simulink model "robot_assembly_backup_oke"  (R2016a)
settings: Solver=VariableStepAuto  StartTime=0.0  StopTime=inf  RelTol=1e-3
values from neighbouring files (symbols this model uses):
  m = size(X, 1)    [polyfitn.m]
undefined symbols (not defined in the file or in its folder): Khop3, Khop_1, Khop_2, Khop_4, Khop_5, Khop_6, robot_assembly, RootGround, RootPart
libraries: mblibv1 x21, simulink x5
settings Model: Creator=Hieu  LastModifiedBy=Hieu
settings GRTTargetCC: GeneratePreprocessorConditionals=Use local settings
settings SimMechanicsCC: VisOnUpdateDiagram=on  VisDuringSimulation=on

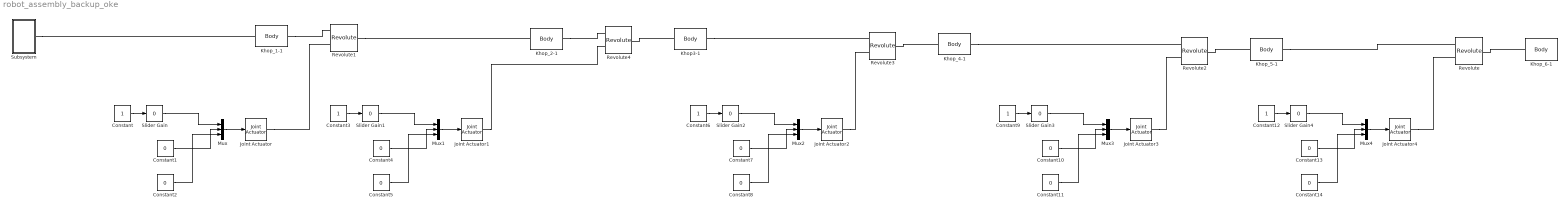
== system robot_assembly_backup_oke ==
  Constant{,3,6,9,12} (5 alike) : Constant
  Constant{1..2,4..5,7..8,10..11,13..14} (10 alike) : Constant  Value=0
  Joint Actuator{,1..4} (5 alike) : mblibv1/Sensors &  Actuators/Joint Actuator  UpdateFromCAD=off  PhysicalDomain=Mechanical  PortType=blob  ActuationStyle=Motion  AngleUnits=deg  ArcVelocityUnits=deg/s  ArcAccelerationUnits=deg/s^2  CoordPositionUnits=m  VelocityUnits=m/s  AccelerationUnits=m/s^2  ForceUnits=N  TorqueUnits=N*m  ActiveIO=on  Width=3  DialogClass=MechanicalActuatorBlock  Primitive=R1  ReferenceFrame=Absolute (World)
  Khop3-1 : mblibv1/Bodies/Body  LConnTagsString=CS3  RConnTagsString=CS2  UpdateFromCAD=on  PMImportedID=Khop3-1  DialogClass=MechanicalBodyBlock  Mass=43.6159  MassUnits=kg  InertiaUnits=kg*m^2  Inertia=[1.17816,2.48356e-09,1.21289e-08;2.48356e-09,0.116751,-0.0778152;1.21289e-08,-0.0778152,1.13755]  Shape=Cylinder  ShapeDims=[1 1]  ShapeUnits=m  ShapeUse=false  Density=1  DensityUnits=kg/m^3  DensityUse=false  GraphicsMode=GFXFILE  GraphicsFileName=robot_assembly - Khop3-1.STL  BodyColorSelMode=COLORPALETTE  BodyColor=[0.776471;0.756863;0.737255]  AttachedToCS=CS1  CG=Right$CG$[0.1867 1.03234 0.317413]$WORLD$WORLD$m$[0.332848 -0.650354 -0.682826;0.890188 0.455594 0;0.311091 -0.607844 0.730581]$3x3 Transform$rad$WORLD$false$Khop3-1::CG(AUTOGEN)  WorkingFrames=Right$CS1$[0.352941 0.944212 0.39173]$WORLD$WORLD$m$[0.332848 -0.650354 -0.682826;0.890188 0.455594 0;0.311091 -0.607844 0.730581]$3x3 Transform$rad$WORLD$false$Khop3-1::CS1(AUTOGEN)#Right$CS2$[-0.028645 1.11825 0.301997]$WORLD$WORLD$m$[1 0 0;0 1 0;0 0 1]$3x3 Transform$rad$WORLD$true$Khop3-1:-:Khop_4-1::Khop3-1(AUTOGEN)#Left$CS3$[0.281245 0.944212 0.468441]$WORLD$WORLD$m$[1 0 0;0 1 0;0 0 1]$3x3 Transform$rad$WORLD$true$Khop3-1:-:Khop_2-1::Khop3-1(AUTOGEN)  CGPos=[0.1867 1.03234 0.317413]  CGRot=[0.332848 -0.650354 -0.682826;0.890188 0.455594 0;0.311091 -0.607844 0.730581]  CS0Pos=[]  CS0Rot=[]  CS1Pos=[0.352941 0.944212 0.39173]  CS1Rot=[0.332848 -0.650354 -0.682826;0.890188 0.455594 0;0.311091 -0.607844 0.730581]  CS2Pos=[-0.028645 1.11825 0.301997]  CS2Rot=[1 0 0;0 1 0;0 0 1]  CS3Pos=[0.281245 0.944212 0.468441]  CS3Rot=[1 0 0;0 1 0;0 0 1]  CS4Pos=[]  CS4Rot=[]  CS5Pos=[]  CS5Rot=[]  CS6Pos=[]  CS6Rot=[]  CS7Pos=[]  CS7Rot=[]  CS8Pos=[]  CS8Rot=[]  CS9Pos=[]  CS9Rot=[]  CS10Pos=[]  CS10Rot=[]  CS11Pos=[]  CS11Rot=[]  CS12Pos=[]  CS12Rot=[]  CS13Pos=[]  CS13Rot=[]  CS14Pos=[]  CS14Rot=[]  CS15Pos=[]  CS15Rot=[]  CS16Pos=[]  CS16Rot=[]  CS17Pos=[]  CS17Rot=[]  CS18Pos=[]  CS18Rot=[]  CS19Pos=[]  CS19Rot=[]  CS20Pos=[]  CS20Rot=[]
  Khop_1-1 : mblibv1/Bodies/Body  LConnTagsString=CS2  RConnTagsString=CS3  UpdateFromCAD=on  PMImportedID=Khop_1-1  DialogClass=MechanicalBodyBlock  Mass=159.648  MassUnits=kg  InertiaUnits=kg*m^2  Inertia=[4.67506,0.0155226,1.62056e-06;0.0155226,1.87752,-4.14461e-06;1.62056e-06,-4.14461e-06,4.39981]  Shape=Cylinder  ShapeDims=[1 1]  ShapeUnits=m  ShapeUse=false  Density=1  DensityUnits=kg/m^3  DensityUse=false  GraphicsMode=GFXFILE  GraphicsFileName=robot_assembly - Khop_1-1.STL  BodyColorSelMode=COLORPALETTE  BodyColor=[0.054902;0.054902;0.054902]  AttachedToCS=CS1  CG=Right$CG$[0.24168 0.390199 0.514197]$WORLD$WORLD$m$[1 0 0;0 1 0;0 0 1]$3x3 Transform$rad$WORLD$false$Khop_1-1::CG(AUTOGEN)  WorkingFrames=Right$CS1$[0.238479 0.145212 0.514197]$WORLD$WORLD$m$[1 0 0;0 1 0;0 0 1]$3x3 Transform$rad$WORLD$false$Khop_1-1::CS1(AUTOGEN)#Left$CS2$[0.24168 0.390199 0.514197]$WORLD$WORLD$m$[1 0 0;0 1 0;0 0 1]$3x3 Transform$rad$WORLD$true$Khop_1-1:-:robot_assembly/RootPart::Khop_1-1(AUTOGEN)#Right$CS3$[0.238479 0.705212 0.514197]$WORLD$WORLD$m$[1 0 0;0 1 0;0 0 1]$3x3 Transform$rad$WORLD$true$Khop_1-1:-:Khop_2-1::Khop_1-1(AUTOGEN)  CGPos=[0.24168 0.390199 0.514197]  CGRot=[1 0 0;0 1 0;0 0 1]  CS0Pos=[]  CS0Rot=[]  CS1Pos=[0.238479 0.145212 0.514197]  CS1Rot=[1 0 0;0 1 0;0 0 1]  CS2Pos=[0.24168 0.390199 0.514197]  CS2Rot=[1 0 0;0 1 0;0 0 1]  CS3Pos=[0.238479 0.705212 0.514197]  CS3Rot=[1 0 0;0 1 0;0 0 1]  CS4Pos=[]  CS4Rot=[]  CS5Pos=[]  CS5Rot=[]  CS6Pos=[]  CS6Rot=[]  CS7Pos=[]  CS7Rot=[]  CS8Pos=[]  CS8Rot=[]  CS9Pos=[]  CS9Rot=[]  CS10Pos=[]  CS10Rot=[]  CS11Pos=[]  CS11Rot=[]  CS12Pos=[]  CS12Rot=[]  CS13Pos=[]  CS13Rot=[]  CS14Pos=[]  CS14Rot=[]  CS15Pos=[]  CS15Rot=[]  CS16Pos=[]  CS16Rot=[]  CS17Pos=[]  CS17Rot=[]  CS18Pos=[]  CS18Rot=[]  CS19Pos=[]  CS19Rot=[]  CS20Pos=[]  CS20Rot=[]
  Khop_2-1 : mblibv1/Bodies/Body  LConnTagsString=CS2  RConnTagsString=CS3  UpdateFromCAD=on  PMImportedID=Khop_2-1  DialogClass=MechanicalBodyBlock  Mass=96.4098  MassUnits=kg  InertiaUnits=kg*m^2  Inertia=[1.36159,-0.133561,-9.98407e-05;-0.133561,0.612029,-6.13842e-05;-9.98407e-05,-6.13842e-05,1.31785]  Shape=Cylinder  ShapeDims=[1 1]  ShapeUnits=m  ShapeUse=false  Density=1  DensityUnits=kg/m^3  DensityUse=false  GraphicsMode=GFXFILE  GraphicsFileName=robot_assembly - Khop_2-1.STL  BodyColorSelMode=COLORPALETTE  BodyColor=[0.94902;0.352941;0.0666667]  AttachedToCS=CS1  CG=Right$CG$[0.224023 0.863366 0.529676]$WORLD$WORLD$m$[-0.682826 0 -0.730581;0 1 0;0.730581 0 -0.682826]$3x3 Transform$rad$WORLD$false$Khop_2-1::CG(AUTOGEN)  WorkingFrames=Right$CS1$[0.238479 0.705212 0.514197]$WORLD$WORLD$m$[-0.682826 0 -0.730581;0 1 0;0.730581 0 -0.682826]$3x3 Transform$rad$WORLD$false$Khop_2-1::CS1(AUTOGEN)#Left$CS2$[0.238479 0.705212 0.514197]$WORLD$WORLD$m$[1 0 0;0 1 0;0 0 1]$3x3 Transform$rad$WORLD$true$Khop_1-1:-:Khop_2-1::Khop_2-1(AUTOGEN)#Right$CS3$[0.281245 0.944212 0.468441]$WORLD$WORLD$m$[1 0 0;0 1 0;0 0 1]$3x3 Transform$rad$WORLD$true$Khop3-1:-:Khop_2-1::Khop_2-1(AUTOGEN)  CGPos=[0.224023 0.863366 0.529676]  CGRot=[-0.682826 0 -0.730581;0 1 0;0.730581 0 -0.682826]  CS0Pos=[]  CS0Rot=[]  CS1Pos=[0.238479 0.705212 0.514197]  CS1Rot=[-0.682826 0 -0.730581;0 1 0;0.730581 0 -0.682826]  CS2Pos=[0.238479 0.705212 0.514197]  CS2Rot=[1 0 0;0 1 0;0 0 1]  CS3Pos=[0.281245 0.944212 0.468441]  CS3Rot=[1 0 0;0 1 0;0 0 1]  CS4Pos=[]  CS4Rot=[]  CS5Pos=[]  CS5Rot=[]  CS6Pos=[]  CS6Rot=[]  CS7Pos=[]  CS7Rot=[]  CS8Pos=[]  CS8Rot=[]  CS9Pos=[]  CS9Rot=[]  CS10Pos=[]  CS10Rot=[]  CS11Pos=[]  CS11Rot=[]  CS12Pos=[]  CS12Rot=[]  CS13Pos=[]  CS13Rot=[]  CS14Pos=[]  CS14Rot=[]  CS15Pos=[]  CS15Rot=[]  CS16Pos=[]  CS16Rot=[]  CS17Pos=[]  CS17Rot=[]  CS18Pos=[]  CS18Rot=[]  CS19Pos=[]  CS19Rot=[]  CS20Pos=[]  CS20Rot=[]
  Khop_4-1 : mblibv1/Bodies/Body  LConnTagsString=CS3  RConnTagsString=CS2  UpdateFromCAD=on  PMImportedID=Khop_4-1  DialogClass=MechanicalBodyBlock  Mass=91.2451  MassUnits=kg  InertiaUnits=kg*m^2  Inertia=[6.24377,0,0.707353;0,6.5607,0;0.707353,0,0.475899]  Shape=Cylinder  ShapeDims=[1 1]  ShapeUnits=m  ShapeUse=false  Density=1  DensityUnits=kg/m^3  DensityUse=false  GraphicsMode=GFXFILE  GraphicsFileName=robot_assembly - Khop_4-1.STL  BodyColorSelMode=COLORPALETTE  BodyColor=[0.776471;0.756863;0.737255]  AttachedToCS=CS1  CG=Right$CG$[-0.127156 1.13763 0.332657]$WORLD$WORLD$m$[-0.682826 0.259349 -0.682998;0 0.93487 0.35499;0.730581 0.242397 -0.638354]$3x3 Transform$rad$WORLD$false$Khop_4-1::CG(AUTOGEN)  WorkingFrames=Right$CS1$[-0.028645 1.11825 0.301997]$WORLD$WORLD$m$[-0.682826 0.259349 -0.682998;0 0.93487 0.35499;0.730581 0.242397 -0.638354]$3x3 Transform$rad$WORLD$false$Khop_4-1::CS1(AUTOGEN)#Right$CS2$[-0.370144 1.29574 -0.0171799]$WORLD$WORLD$m$[1 0 0;0 1 0;0 0 1]$3x3 Transform$rad$WORLD$true$Khop_4-1:-:Khop_5-1::Khop_4-1(AUTOGEN)#Left$CS3$[-0.028645 1.11825 0.301997]$WORLD$WORLD$m$[1 0 0;0 1 0;0 0 1]$3x3 Transform$rad$WORLD$true$Khop3-1:-:Khop_4-1::Khop_4-1(AUTOGEN)  CGPos=[-0.127156 1.13763 0.332657]  CGRot=[-0.682826 0.259349 -0.682998;0 0.93487 0.35499;0.730581 0.242397 -0.638354]  CS0Pos=[]  CS0Rot=[]  CS1Pos=[-0.028645 1.11825 0.301997]  CS1Rot=[-0.682826 0.259349 -0.682998;0 0.93487 0.35499;0.730581 0.242397 -0.638354]  CS2Pos=[-0.370144 1.29574 -0.0171799]  CS2Rot=[1 0 0;0 1 0;0 0 1]  CS3Pos=[-0.028645 1.11825 0.301997]  CS3Rot=[1 0 0;0 1 0;0 0 1]  CS4Pos=[]  CS4Rot=[]  CS5Pos=[]  CS5Rot=[]  CS6Pos=[]  CS6Rot=[]  CS7Pos=[]  CS7Rot=[]  CS8Pos=[]  CS8Rot=[]  CS9Pos=[]  CS9Rot=[]  CS10Pos=[]  CS10Rot=[]  CS11Pos=[]  CS11Rot=[]  CS12Pos=[]  CS12Rot=[]  CS13Pos=[]  CS13Rot=[]  CS14Pos=[]  CS14Rot=[]  CS15Pos=[]  CS15Rot=[]  CS16Pos=[]  CS16Rot=[]  CS17Pos=[]  CS17Rot=[]  CS18Pos=[]  CS18Rot=[]  CS19Pos=[]  CS19Rot=[]  CS20Pos=[]  CS20Rot=[]
  Khop_5-1 : mblibv1/Bodies/Body  LConnTagsString=CS3  RConnTagsString=CS2  UpdateFromCAD=on  PMImportedID=Khop_5-1  DialogClass=MechanicalBodyBlock  Mass=4.20495  MassUnits=kg  InertiaUnits=kg*m^2  Inertia=[0.00605149,-7.30355e-05,-2.13324e-09;-7.30355e-05,0.00377876,2.04521e-09;-2.13324e-09,2.04521e-09,0.00491242]  Shape=Cylinder  ShapeDims=[1 1]  ShapeUnits=m  ShapeUse=false  Density=1  DensityUnits=kg/m^3  DensityUse=false  GraphicsMode=GFXFILE  GraphicsFileName=robot_assembly - Khop_5-1.STL  BodyColorSelMode=COLORPALETTE  BodyColor=[0.776471;0.756863;0.737255]  AttachedToCS=CS1  CG=Right$CG$[-0.350069 1.29118 -0.0409774]$WORLD$WORLD$m$[-0.682826 -0.239308 0.690275;0 -0.944831 -0.327558;0.730581 -0.223665 0.645156]$3x3 Transform$rad$WORLD$false$Khop_5-1::CG(AUTOGEN)  WorkingFrames=Right$CS1$[-0.332589 1.29574 -0.0573619]$WORLD$WORLD$m$[-0.682826 -0.239308 0.690275;0 -0.944831 -0.327558;0.730581 -0.223665 0.645156]$3x3 Transform$rad$WORLD$false$Khop_5-1::CS1(AUTOGEN)#Right$CS2$[-0.363332 1.2485 -0.0484542]$WORLD$WORLD$m$[1 0 0;0 1 0;0 0 1]$3x3 Transform$rad$WORLD$true$Khop_5-1:-:Khop_6-1::Khop_5-1(AUTOGEN)#Left$CS3$[-0.370144 1.29574 -0.0171799]$WORLD$WORLD$m$[1 0 0;0 1 0;0 0 1]$3x3 Transform$rad$WORLD$true$Khop_4-1:-:Khop_5-1::Khop_5-1(AUTOGEN)  CGPos=[-0.350069 1.29118 -0.0409774]  CGRot=[-0.682826 -0.239308 0.690275;0 -0.944831 -0.327558;0.730581 -0.223665 0.645156]  CS0Pos=[]  CS0Rot=[]  CS1Pos=[-0.332589 1.29574 -0.0573619]  CS1Rot=[-0.682826 -0.239308 0.690275;0 -0.944831 -0.327558;0.730581 -0.223665 0.645156]  CS2Pos=[-0.363332 1.2485 -0.0484542]  CS2Rot=[1 0 0;0 1 0;0 0 1]  CS3Pos=[-0.370144 1.29574 -0.0171799]  CS3Rot=[1 0 0;0 1 0;0 0 1]  CS4Pos=[]  CS4Rot=[]  CS5Pos=[]  CS5Rot=[]  CS6Pos=[]  CS6Rot=[]  CS7Pos=[]  CS7Rot=[]  CS8Pos=[]  CS8Rot=[]  CS9Pos=[]  CS9Rot=[]  CS10Pos=[]  CS10Rot=[]  CS11Pos=[]  CS11Rot=[]  CS12Pos=[]  CS12Rot=[]  CS13Pos=[]  CS13Rot=[]  CS14Pos=[]  CS14Rot=[]  CS15Pos=[]  CS15Rot=[]  CS16Pos=[]  CS16Rot=[]  CS17Pos=[]  CS17Rot=[]  CS18Pos=[]  CS18Rot=[]  CS19Pos=[]  CS19Rot=[]  CS20Pos=[]  CS20Rot=[]
  Khop_6-1 : mblibv1/Bodies/Body  LConnTagsString=CS2  UpdateFromCAD=on  PMImportedID=Khop_6-1  DialogClass=MechanicalBodyBlock  Mass=0.0714507  MassUnits=kg  InertiaUnits=kg*m^2  Inertia=[3.56662e-05,1.85941e-09,1.77541e-10;1.85941e-09,5.05769e-05,2.11404e-10;1.77541e-10,2.11404e-10,2.23778e-05]  Shape=Cylinder  ShapeDims=[1 1]  ShapeUnits=m  ShapeUse=false  Density=1  DensityUnits=kg/m^3  DensityUse=false  GraphicsMode=GFXFILE  GraphicsFileName=robot_assembly - Khop_6-1.STL  BodyColorSelMode=COLORPALETTE  BodyColor=[0.792157;0.819608;0.933333]  AttachedToCS=CS1  CG=Right$CG$[-0.372928 1.21061 -0.0574269]$WORLD$WORLD$m$[-0.0811385 0.239308 0.967548;0.249013 0.944831 -0.212807;-0.965095 0.223665 -0.136253]$3x3 Transform$rad$WORLD$false$Khop_6-1::CG(AUTOGEN)  WorkingFrames=Right$CS1$[-0.369314 1.22488 -0.0540458]$WORLD$WORLD$m$[-0.0811385 0.239308 0.967548;0.249013 0.944831 -0.212807;-0.965095 0.223665 -0.136253]$3x3 Transform$rad$WORLD$false$Khop_6-1::CS1(AUTOGEN)#Left$CS2$[-0.363332 1.2485 -0.0484542]$WORLD$WORLD$m$[1 0 0;0 1 0;0 0 1]$3x3 Transform$rad$WORLD$true$Khop_5-1:-:Khop_6-1::Khop_6-1(AUTOGEN)  CGPos=[-0.372928 1.21061 -0.0574269]  CGRot=[-0.0811385 0.239308 0.967548;0.249013 0.944831 -0.212807;-0.965095 0.223665 -0.136253]  CS0Pos=[]  CS0Rot=[]  CS1Pos=[-0.369314 1.22488 -0.0540458]  CS1Rot=[-0.0811385 0.239308 0.967548;0.249013 0.944831 -0.212807;-0.965095 0.223665 -0.136253]  CS2Pos=[-0.363332 1.2485 -0.0484542]  CS2Rot=[1 0 0;0 1 0;0 0 1]  CS3Pos=[]  CS3Rot=[]  CS4Pos=[]  CS4Rot=[]  CS5Pos=[]  CS5Rot=[]  CS6Pos=[]  CS6Rot=[]  CS7Pos=[]  CS7Rot=[]  CS8Pos=[]  CS8Rot=[]  CS9Pos=[]  CS9Rot=[]  CS10Pos=[]  CS10Rot=[]  CS11Pos=[]  CS11Rot=[]  CS12Pos=[]  CS12Rot=[]  CS13Pos=[]  CS13Rot=[]  CS14Pos=[]  CS14Rot=[]  CS15Pos=[]  CS15Rot=[]  CS16Pos=[]  CS16Rot=[]  CS17Pos=[]  CS17Rot=[]  CS18Pos=[]  CS18Rot=[]  CS19Pos=[]  CS19Rot=[]  CS20Pos=[]  CS20Rot=[]
  Mux{,1..4} (5 alike) : Mux  Inputs=3
  Revolute : mblibv1/Joints/Revolute  LConnTagsString=__newl0|SA1  RConnTagsString=__newr0  UpdateFromCAD=on  PMImportedID=Khop_5-1:-:Khop_6-1  NumSAPorts=1  CutJoint=off  MarkAsCut=off  Primitives=prismatic  PrimitiveProps=R1$World$[0.239308,0.944831,0.223665]$revolute  DialogClass=JointBlock  R1Axis=[0.239308,0.944831,0.223665]
  Revolute1 : mblibv1/Joints/Revolute  LConnTagsString=__newl0|SA1  RConnTagsString=__newr0  UpdateFromCAD=on  PMImportedID=Khop_1-1:-:Khop_2-1  NumSAPorts=1  CutJoint=off  MarkAsCut=off  Primitives=prismatic  PrimitiveProps=R1$World$[0,1,0]$revolute  DialogClass=JointBlock  R1Axis=[0,1,0]
  Revolute2 : mblibv1/Joints/Revolute  LConnTagsString=__newl0|SA1  RConnTagsString=__newr0  UpdateFromCAD=on  PMImportedID=Khop_4-1:-:Khop_5-1  NumSAPorts=1  CutJoint=off  MarkAsCut=off  Primitives=prismatic  PrimitiveProps=R1$World$[0.682826,0,-0.730581]$revolute  DialogClass=JointBlock  R1Axis=[0.682826,0,-0.730581]
  Revolute3 : mblibv1/Joints/Revolute  LConnTagsString=__newl0|SA1  RConnTagsString=__newr0  UpdateFromCAD=on  PMImportedID=Khop3-1:-:Khop_4-1  NumSAPorts=1  CutJoint=off  MarkAsCut=off  Primitives=prismatic  PrimitiveProps=R1$World$[-0.682826,0,0.730581]$revolute  DialogClass=JointBlock  R1Axis=[-0.682826,0,0.730581]
  Revolute4 : mblibv1/Joints/Revolute  LConnTagsString=__newl0|SA1  RConnTagsString=__newr0  UpdateFromCAD=on  PMImportedID=Khop3-1:-:Khop_2-1  NumSAPorts=1  CutJoint=off  MarkAsCut=off  Primitives=prismatic  PrimitiveProps=R1$World$[-0.682826,0,0.730581]$revolute  DialogClass=JointBlock  R1Axis=[-0.682826,0,0.730581]
  Slider Gain{,1..4} (5 alike) : simulink/Math Operations/Slider Gain  low=-180  gain=0  high=180
  Subsystem : Subsystem
  wires:
  Slider Gain/1 -> Mux/1
  Constant1/1 -> Mux/2
  Constant2/1 -> Mux/3
  Constant/1 -> Slider Gain/1
  Mux/1 -> Joint Actuator/1
  Slider Gain1/1 -> Mux1/1
  Constant4/1 -> Mux1/2
  Constant5/1 -> Mux1/3
  Constant3/1 -> Slider Gain1/1
  Mux1/1 -> Joint Actuator1/1
  Slider Gain2/1 -> Mux2/1
  Constant7/1 -> Mux2/2
  Constant8/1 -> Mux2/3
  Constant6/1 -> Slider Gain2/1
  Mux2/1 -> Joint Actuator2/1
  Slider Gain3/1 -> Mux3/1
  Constant10/1 -> Mux3/2
  Constant11/1 -> Mux3/3
  Constant9/1 -> Slider Gain3/1
  Mux3/1 -> Joint Actuator3/1
  Slider Gain4/1 -> Mux4/1
  Constant13/1 -> Mux4/2
  Constant14/1 -> Mux4/3
  Constant12/1 -> Slider Gain4/1
  Mux4/1 -> Joint Actuator4/1
  connections:
  Khop_5-1/RConn1 -- Revolute/LConn1
  Revolute/RConn1 -- Khop_6-1/LConn1
  Khop_1-1/RConn1 -- Revolute1/LConn1
  Revolute1/RConn1 -- Khop_2-1/LConn1
  Khop_4-1/RConn1 -- Revolute2/LConn1
  Revolute2/RConn1 -- Khop_5-1/LConn1
  Khop3-1/RConn1 -- Revolute3/LConn1
  Revolute3/RConn1 -- Khop_4-1/LConn1
  Khop_2-1/RConn1 -- Revolute4/LConn1
  Revolute4/RConn1 -- Khop3-1/LConn1
  Subsystem/RConn1 -- Khop_1-1/LConn1
  Joint Actuator/RConn1 -- Revolute1/LConn2
  Joint Actuator1/RConn1 -- Revolute4/LConn2
  Joint Actuator2/RConn1 -- Revolute3/LConn2
  Joint Actuator3/RConn1 -- Revolute2/LConn2
  Joint Actuator4/RConn1 -- Revolute/LConn2

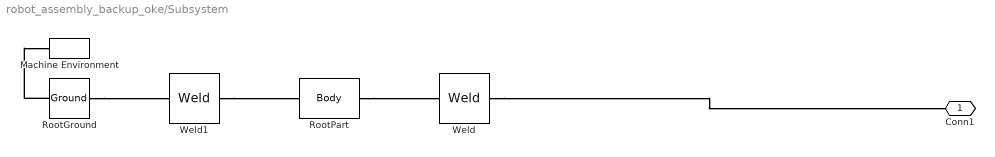
== system robot_assembly_backup_oke/Subsystem ==
  Machine Environment : mblibv1/Bodies/Machine Environment  PortType=env  PhysicalDomain=Mechanical  DialogTemplateClass=MECH.MachineEnvironment  SyncWhenCopied=off  Gravity=[0 -9.81 0]  GravityUnits=m/s^2  GravityAsSignal=off  Dimensionality=Auto-detect  AnalysisType=Forward dynamics  LinearAssemblyTolerance=1e-3  LinearAssemblyToleranceUnits=m  AngularAssemblyTolerance=1e-3  AngularAssemblyToleranceUnits=rad  ConstraintSolverType=Stabilizing  ConstraintRelTolerance=1e-4  ConstraintAbsTolerance=1e-4  UseRobustSingularityHandling=off  RedundancyAnalysisToleranceType=Automatically select tolerance  RedundancyAnalysisTolerance=1e-14  StatePerturbationType=Fixed  PerturbationSize=1e-5  VisualizeMachine=on  BodyVisualizationType=Use model default body geometries  BodyColorSelMode=Use model default  DefaultBodyColor=[1 0 0]
  RootGround : mblibv1/Bodies/Ground  UpdateFromCAD=on  PMImportedID=RootGround  LeftPortType=env  RightPortType=workingframe  PhysicalDomain=Mechanical  DialogClass=GroundBlock  CoordPosition=[0.139738,0.758807,0.44833]  CoordPositionUnits=m  StateVectorMgrId=2  MachineId=[2 0]  ShowEnvPort=on  ParameterChecksum=[1012169240, 3549377625, 1504519537, 2767636779]  TopologyChecksum=[3745075106, 3381574792, 3677716977, 1012078593]
  RootPart : mblibv1/Bodies/Body  LConnTagsString=CS3  RConnTagsString=CS2  UpdateFromCAD=on  PMImportedID=robot_assembly/RootPart  DialogClass=MechanicalBodyBlock  Mass=0  MassUnits=kg  InertiaUnits=kg*m^2  Inertia=[0,0,0;0,0,0;0,0,0]  Shape=Cylinder  ShapeDims=[1 1]  ShapeUnits=m  ShapeUse=false  Density=1  DensityUnits=kg/m^3  DensityUse=false  GraphicsMode=MACHINE_DEFAULT  BodyColorSelMode=MACHINE_DEFAULT  BodyColor=[1;0;0]  AttachedToCS=CS1  CG=Right$CG$[0.139738 0.758807 0.44833]$WORLD$WORLD$m$[1 0 0;0 1 0;0 0 1]$3x3 Transform$rad$WORLD$false$robot_assembly/RootPart::CG(AUTOGEN)  WorkingFrames=Right$CS1$[0 0 0]$WORLD$WORLD$m$[1 0 0;0 1 0;0 0 1]$3x3 Transform$rad$WORLD$false$robot_assembly/RootPart::CS1(AUTOGEN)#Right$CS2$[0.24168 0.390199 0.514197]$WORLD$WORLD$m$[1 0 0;0 1 0;0 0 1]$3x3 Transform$rad$WORLD$true$Khop_1-1:-:robot_assembly/RootPart::robot_assembly/RootPart(AUTOGEN)#Left$CS3$[0.139738 0.758807 0.44833]$WORLD$WORLD$m$[1 0 0;0 1 0;0 0 1]$3x3 Transform$rad$WORLD$true$RootGround:-:robot_assembly/RootPart::robot_assembly/RootPart(AUTOGEN)  CGPos=[0.139738 0.758807 0.44833]  CGRot=[1 0 0;0 1 0;0 0 1]  CS0Pos=[]  CS0Rot=[]  CS1Pos=[0 0 0]  CS1Rot=[1 0 0;0 1 0;0 0 1]  CS2Pos=[0.24168 0.390199 0.514197]  CS2Rot=[1 0 0;0 1 0;0 0 1]  CS3Pos=[0.139738 0.758807 0.44833]  CS3Rot=[1 0 0;0 1 0;0 0 1]  CS4Pos=[]  CS4Rot=[]  CS5Pos=[]  CS5Rot=[]  CS6Pos=[]  CS6Rot=[]  CS7Pos=[]  CS7Rot=[]  CS8Pos=[]  CS8Rot=[]  CS9Pos=[]  CS9Rot=[]  CS10Pos=[]  CS10Rot=[]  CS11Pos=[]  CS11Rot=[]  CS12Pos=[]  CS12Rot=[]  CS13Pos=[]  CS13Rot=[]  CS14Pos=[]  CS14Rot=[]  CS15Pos=[]  CS15Rot=[]  CS16Pos=[]  CS16Rot=[]  CS17Pos=[]  CS17Rot=[]  CS18Pos=[]  CS18Rot=[]  CS19Pos=[]  CS19Rot=[]  CS20Pos=[]  CS20Rot=[]
  Weld : mblibv1/Joints/Weld  LConnTagsString=__newl0  RConnTagsString=__newr0  UpdateFromCAD=on  PMImportedID=Khop_1-1:-:robot_assembly/RootPart  NumSAPorts=0  CutJoint=off  MarkAsCut=off  Primitives=weld  PrimitiveProps=W$WORLD$[0.57735,0.57735,0.57735]$weld  DialogClass=JointBlock  WAxis=[0.57735,0.57735,0.57735]
  Weld1 : mblibv1/Joints/Weld  LConnTagsString=__newl0  RConnTagsString=__newr0  UpdateFromCAD=on  PMImportedID=RootGround:-:robot_assembly/RootPart  NumSAPorts=0  CutJoint=off  MarkAsCut=off  Primitives=weld  PrimitiveProps=W$WORLD$[0.57735,0.57735,0.57735]$weld  DialogClass=JointBlock  WAxis=[0.57735,0.57735,0.57735]
  Conn1 : PMIOPort  Port=1  Side=Right
  connections:
  RootGround/RConn1 -- Weld1/LConn1
  Weld1/RConn1 -- RootPart/LConn1
  RootGround/LConn1 -- Machine Environment/RConn1
  Weld/RConn1 -- Conn1/RConn1
  RootPart/RConn1 -- Weld/LConn1
